simulink model "untitled1"  (R2018a)
settings: Solver=FixedStepAuto  StartTime=0.0  StopTime=2500  RelTol=1e-3
settings Model: Creator=johnb  LastModifiedBy=johnb

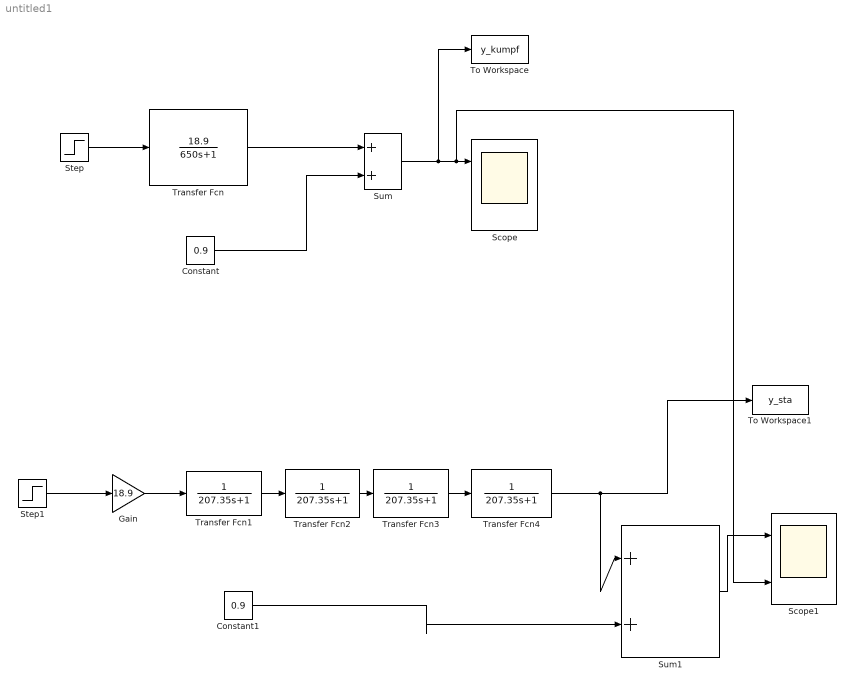
== system untitled1 ==
  Constant : Constant  Value=0.9
  Constant1 : Constant  Value=0.9
  Gain : Gain  Gain=18.9
  Scope : Scope  NumInputPorts=2
  Scope1 : Scope  NumInputPorts=2
  Step : Step  Time=225  SampleTime=0
  Step1 : Step  Time=17.65  SampleTime=0
  Sum : Sum  Inputs=2
  Sum1 : Sum  Inputs=|++
  To Workspace : ToWorkspace  VariableName=y_kumpf  SaveFormat=Timeseries  SampleTime=-1
  To Workspace1 : ToWorkspace  VariableName=y_sta  SaveFormat=Timeseries  SampleTime=-1
  Transfer Fcn : TransferFcn  Numerator=[18.9]  Denominator=[650 1]
  Transfer Fcn{1..4} (4 alike) : TransferFcn  Denominator=[207.35 1]
  wires:
  Step/1 -> Transfer Fcn/1
  Constant/1 -> Sum/2
  Transfer Fcn/1 -> Sum/1
  Sum/1 -> To Workspace/1, Scope1/2, Scope/1
  Step1/1 -> Gain/1
  Transfer Fcn3/1 -> Transfer Fcn4/1
  Transfer Fcn1/1 -> Transfer Fcn2/1
  Transfer Fcn2/1 -> Transfer Fcn3/1
  Gain/1 -> Transfer Fcn1/1
  Transfer Fcn4/1 -> Sum1/1, To Workspace1/1
  Constant1/1 -> Sum1/2
  Sum1/1 -> Scope1/1
